simulink model "RC_Logitech_Mac"  (R2017b)
settings: Solver=FixedStepDiscrete  StartTime=0.0  StopTime=inf  RelTol=1e-3
libraries: vrlib x1
settings Model: Creator=zht  LastModifiedBy=zht

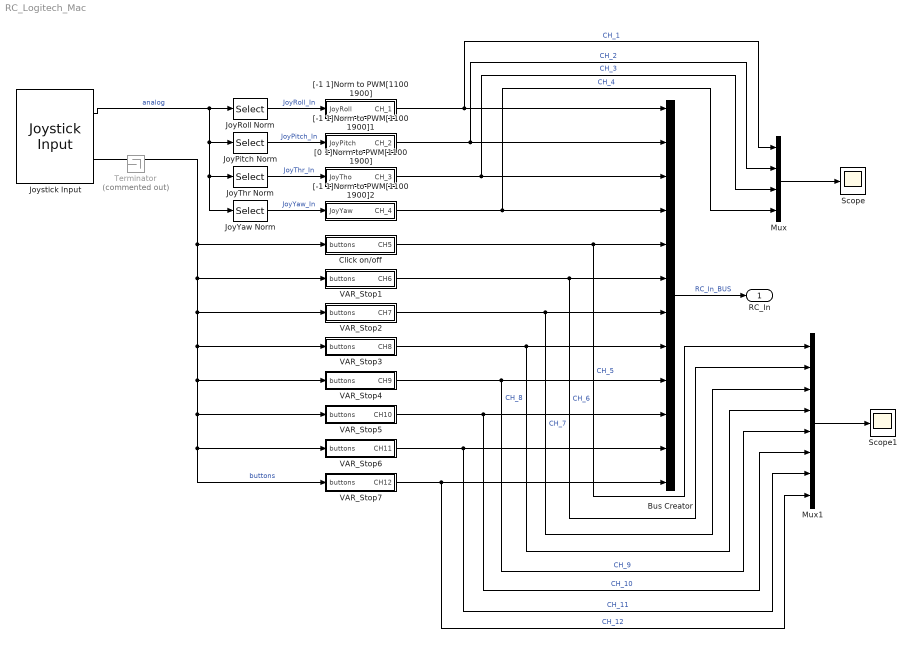
== system RC_Logitech_Mac ==
  Bus Creator : BusCreator  Inputs=12  OutDataTypeStr=Bus: RC_In_BUS  NonVirtualBus=on
  Click on/off : Subsystem
  JoyPitch Norm : Selector  InputPortWidth=4  IndexOptions=Index vector (dialog)  Indices=[2]  OutputSizes=1
  JoyRoll Norm : Selector  InputPortWidth=4  IndexOptions=Index vector (dialog)  Indices=[1]  OutputSizes=1
  JoyThr Norm : Selector  InputPortWidth=4  IndexOptions=Index vector (dialog)  Indices=[4]  OutputSizes=1
  JoyYaw Norm : Selector  InputPortWidth=4  IndexOptions=Index vector (dialog)  Indices=[3]  OutputSizes=1
  Joystick Input : vrlib/Joystick Input  joyid=1  adjustports=on  forcefeed=off
      settings: SourceProductBaseCode=VR
  Mux : Mux
  Mux1 : Mux  Inputs=8
  Scope : Scope
  Scope1 : Scope
  Terminator : Terminator  Commented=on
  VAR_Stop1 : Subsystem
  VAR_Stop2 : Subsystem
  VAR_Stop3 : Subsystem
  VAR_Stop4 : Subsystem
  VAR_Stop5 : Subsystem
  VAR_Stop6 : Subsystem
  VAR_Stop7 : Subsystem
  "[-1 1]Norm to PWM[1100 1900]" : Subsystem
  "[-1 1]Norm to PWM[1100 1900]1" : Subsystem
  "[-1 1]Norm to PWM[1100 1900]2" : Subsystem
  "[0 1]Norm to PWM[1100 1900]" : Subsystem
  RC_In : Outport  OutDataTypeStr=Bus: RC_In_BUS
  wires:
  Bus Creator/1 -> RC_In/1  "RC_In_BUS"
  JoyYaw Norm/1 -> "[-1 1]Norm to PWM[1100 1900]2"/1(JoyYaw)  "JoyYaw_In"
  JoyPitch Norm/1 -> "[-1 1]Norm to PWM[1100 1900]1"/1(JoyPitch)  "JoyPitch_In"
  "[0 1]Norm to PWM[1100 1900]"/1(CH_3) -> Bus Creator/3, Mux/3  "CH_3"
  Joystick Input/2 -> Click on/off/1(buttons), VAR_Stop1/1(buttons), VAR_Stop2/1(buttons), VAR_Stop3/1(buttons), VAR_Stop5/1(buttons), VAR_Stop6/1(buttons), VAR_Stop7/1(buttons), VAR_Stop4/1(buttons)  "buttons"
  Joystick Input/1 -> JoyYaw Norm/1, JoyThr Norm/1, JoyPitch Norm/1, JoyRoll Norm/1  "analog"
  "[-1 1]Norm to PWM[1100 1900]1"/1(CH_2) -> Bus Creator/2, Mux/2  "CH_2"
  "[-1 1]Norm to PWM[1100 1900]"/1(CH_1) -> Bus Creator/1, Mux/1  "CH_1"
  JoyThr Norm/1 -> "[0 1]Norm to PWM[1100 1900]"/1(JoyTho)  "JoyThr_In"
  JoyRoll Norm/1 -> "[-1 1]Norm to PWM[1100 1900]"/1(JoyRoll)  "JoyRoll_In"
  "[-1 1]Norm to PWM[1100 1900]2"/1(CH_4) -> Bus Creator/4, Mux/4  "CH_4"
  Click on/off/1(CH5) -> Bus Creator/5, Mux1/1  "CH_5"
  VAR_Stop1/1(CH6) -> Bus Creator/6, Mux1/2  "CH_6"
  VAR_Stop2/1(CH7) -> Bus Creator/7, Mux1/3  "CH_7"
  VAR_Stop3/1(CH8) -> Bus Creator/8, Mux1/4  "CH_8"
  VAR_Stop4/1(CH9) -> Bus Creator/9, Mux1/5  "CH_9"
  VAR_Stop5/1(CH10) -> Bus Creator/10, Mux1/6  "CH_10"
  VAR_Stop6/1(CH11) -> Bus Creator/11, Mux1/7  "CH_11"
  VAR_Stop7/1(CH12) -> Bus Creator/12, Mux1/8  "CH_12"
  Mux/1 -> Scope/1
  Mux1/1 -> Scope1/1

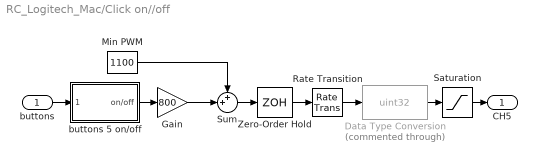
== system RC_Logitech_Mac/Click on//off ==
  buttons : Inport
  Data Type Conversion : DataTypeConversion  Commented=through  OutDataTypeStr=uint32
  Gain : Gain  Gain=800
  Min PWM : Constant  Value=1100
  Rate Transition : RateTransition
  Saturation : Saturate  UpperLimit=1900  LowerLimit=1100
  Sum : Sum  Inputs=++|
  Zero-Order Hold : ZeroOrderHold  SampleTime=0.02
  buttons 5 on/off : Subsystem
  CH5 : Outport
  wires:
  buttons/1 -> buttons 5 on/off/1(buttons)
  Min PWM/1 -> Sum/1
  Rate Transition/1 -> Data Type Conversion/1
  buttons 5 on/off/1(on/off) -> Gain/1
  Gain/1 -> Sum/2
  Data Type Conversion/1 -> Saturation/1
  Sum/1 -> Zero-Order Hold/1
  Zero-Order Hold/1 -> Rate Transition/1
  Saturation/1 -> CH5/1

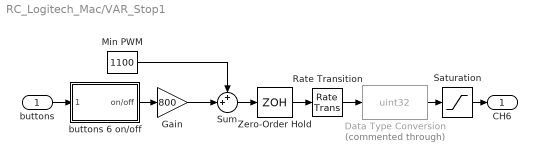
== system RC_Logitech_Mac/VAR_Stop1 ==
  buttons : Inport
  Data Type Conversion : DataTypeConversion  Commented=through  OutDataTypeStr=uint32
  Gain : Gain  Gain=800
  Min PWM : Constant  Value=1100
  Rate Transition : RateTransition
  Saturation : Saturate  UpperLimit=1900  LowerLimit=1100
  Sum : Sum  Inputs=++|
  Zero-Order Hold : ZeroOrderHold  SampleTime=0.02
  buttons 6 on/off : Subsystem
  CH6 : Outport
  wires:
  Saturation/1 -> CH6/1
  Zero-Order Hold/1 -> Rate Transition/1
  Sum/1 -> Zero-Order Hold/1
  Data Type Conversion/1 -> Saturation/1
  Gain/1 -> Sum/2
  buttons 6 on/off/1(on/off) -> Gain/1
  Rate Transition/1 -> Data Type Conversion/1
  Min PWM/1 -> Sum/1
  buttons/1 -> buttons 6 on/off/1(buttons)

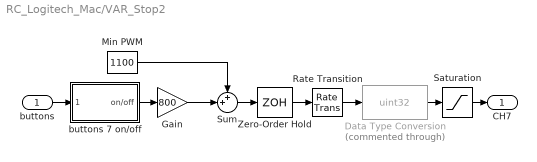
== system RC_Logitech_Mac/VAR_Stop2 ==
  buttons : Inport
  Data Type Conversion : DataTypeConversion  Commented=through  OutDataTypeStr=uint32
  Gain : Gain  Gain=800
  Min PWM : Constant  Value=1100
  Rate Transition : RateTransition
  Saturation : Saturate  UpperLimit=1900  LowerLimit=1100
  Sum : Sum  Inputs=++|
  Zero-Order Hold : ZeroOrderHold  SampleTime=0.02
  buttons 7 on/off : Subsystem
  CH7 : Outport
  wires:
  buttons/1 -> buttons 7 on/off/1(buttons)
  Min PWM/1 -> Sum/1
  Rate Transition/1 -> Data Type Conversion/1
  buttons 7 on/off/1(on/off) -> Gain/1
  Gain/1 -> Sum/2
  Data Type Conversion/1 -> Saturation/1
  Sum/1 -> Zero-Order Hold/1
  Zero-Order Hold/1 -> Rate Transition/1
  Saturation/1 -> CH7/1

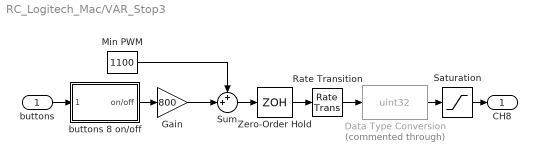
== system RC_Logitech_Mac/VAR_Stop3 ==
  buttons : Inport
  Data Type Conversion : DataTypeConversion  Commented=through  OutDataTypeStr=uint32
  Gain : Gain  Gain=800
  Min PWM : Constant  Value=1100
  Rate Transition : RateTransition
  Saturation : Saturate  UpperLimit=1900  LowerLimit=1100
  Sum : Sum  Inputs=++|
  Zero-Order Hold : ZeroOrderHold  SampleTime=0.02
  buttons 8 on/off : Subsystem
  CH8 : Outport
  wires:
  Saturation/1 -> CH8/1
  Zero-Order Hold/1 -> Rate Transition/1
  Sum/1 -> Zero-Order Hold/1
  Data Type Conversion/1 -> Saturation/1
  Gain/1 -> Sum/2
  buttons 8 on/off/1(on/off) -> Gain/1
  Rate Transition/1 -> Data Type Conversion/1
  Min PWM/1 -> Sum/1
  buttons/1 -> buttons 8 on/off/1(buttons)

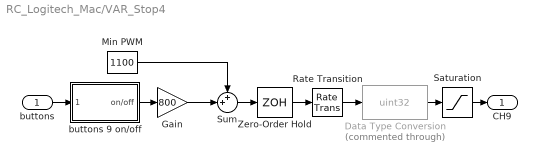
== system RC_Logitech_Mac/VAR_Stop4 ==
  buttons : Inport
  Data Type Conversion : DataTypeConversion  Commented=through  OutDataTypeStr=uint32
  Gain : Gain  Gain=800
  Min PWM : Constant  Value=1100
  Rate Transition : RateTransition
  Saturation : Saturate  UpperLimit=1900  LowerLimit=1100
  Sum : Sum  Inputs=++|
  Zero-Order Hold : ZeroOrderHold  SampleTime=0.02
  buttons 9 on/off : Subsystem
  CH9 : Outport
  wires:
  buttons/1 -> buttons 9 on/off/1(buttons)
  Min PWM/1 -> Sum/1
  Rate Transition/1 -> Data Type Conversion/1
  buttons 9 on/off/1(on/off) -> Gain/1
  Gain/1 -> Sum/2
  Data Type Conversion/1 -> Saturation/1
  Sum/1 -> Zero-Order Hold/1
  Zero-Order Hold/1 -> Rate Transition/1
  Saturation/1 -> CH9/1

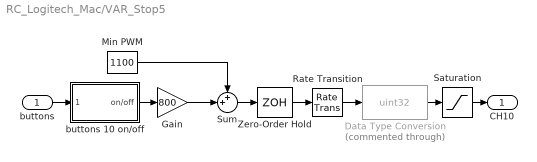
== system RC_Logitech_Mac/VAR_Stop5 ==
  buttons : Inport
  Data Type Conversion : DataTypeConversion  Commented=through  OutDataTypeStr=uint32
  Gain : Gain  Gain=800
  Min PWM : Constant  Value=1100
  Rate Transition : RateTransition
  Saturation : Saturate  UpperLimit=1900  LowerLimit=1100
  Sum : Sum  Inputs=++|
  Zero-Order Hold : ZeroOrderHold  SampleTime=0.02
  buttons 10 on/off : Subsystem
  CH10 : Outport
  wires:
  Saturation/1 -> CH10/1
  Zero-Order Hold/1 -> Rate Transition/1
  Sum/1 -> Zero-Order Hold/1
  Data Type Conversion/1 -> Saturation/1
  Gain/1 -> Sum/2
  buttons 10 on/off/1(on/off) -> Gain/1
  Rate Transition/1 -> Data Type Conversion/1
  Min PWM/1 -> Sum/1
  buttons/1 -> buttons 10 on/off/1(buttons)

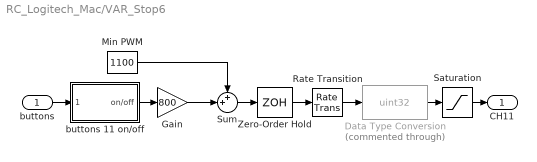
== system RC_Logitech_Mac/VAR_Stop6 ==
  buttons : Inport
  Data Type Conversion : DataTypeConversion  Commented=through  OutDataTypeStr=uint32
  Gain : Gain  Gain=800
  Min PWM : Constant  Value=1100
  Rate Transition : RateTransition
  Saturation : Saturate  UpperLimit=1900  LowerLimit=1100
  Sum : Sum  Inputs=++|
  Zero-Order Hold : ZeroOrderHold  SampleTime=0.02
  buttons 11 on/off : Subsystem
  CH11 : Outport
  wires:
  buttons/1 -> buttons 11 on/off/1(buttons)
  Min PWM/1 -> Sum/1
  Rate Transition/1 -> Data Type Conversion/1
  buttons 11 on/off/1(on/off) -> Gain/1
  Gain/1 -> Sum/2
  Data Type Conversion/1 -> Saturation/1
  Sum/1 -> Zero-Order Hold/1
  Zero-Order Hold/1 -> Rate Transition/1
  Saturation/1 -> CH11/1

== system RC_Logitech_Mac/VAR_Stop7 ==
  buttons : Inport
  Data Type Conversion : DataTypeConversion  Commented=through  OutDataTypeStr=uint32
  Gain : Gain  Gain=800
  Min PWM : Constant  Value=1100
  Rate Transition : RateTransition
  Saturation : Saturate  UpperLimit=1900  LowerLimit=1100
  Sum : Sum  Inputs=++|
  Zero-Order Hold : ZeroOrderHold  SampleTime=0.02
  buttons 12 on/off : Subsystem
  CH12 : Outport
  wires:
  Saturation/1 -> CH12/1
  Zero-Order Hold/1 -> Rate Transition/1
  Sum/1 -> Zero-Order Hold/1
  Data Type Conversion/1 -> Saturation/1
  Gain/1 -> Sum/2
  buttons 12 on/off/1(on/off) -> Gain/1
  Rate Transition/1 -> Data Type Conversion/1
  Min PWM/1 -> Sum/1
  buttons/1 -> buttons 12 on/off/1(buttons)

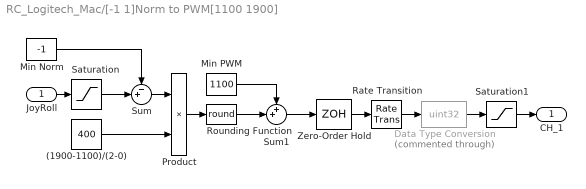
== system RC_Logitech_Mac/[-1 1]Norm to PWM[1100 1900] ==
  JoyRoll : Inport  OutDataTypeStr=double  Unit=1  PortDimensions=1
  (1900-1100)/(2-0) : Constant  Value=400  OutDataTypeStr=uint32
  Data Type Conversion : DataTypeConversion  Commented=through  OutDataTypeStr=uint32
  Min Norm : Constant  Value=-1
  Min PWM : Constant  Value=1100  OutDataTypeStr=uint32
  Product : Product  Inputs=**
  Rate Transition : RateTransition
  Rounding Function : Rounding  Operator=round
  Saturation : Saturate  UpperLimit=1  LowerLimit=-1
  Saturation1 : Saturate  UpperLimit=1900  LowerLimit=1100
  Sum : Sum  Inputs=-+|
  Sum1 : Sum  Inputs=++|
  Zero-Order Hold : ZeroOrderHold  SampleTime=0.02
  CH_1 : Outport  OutMin=[1100]  OutMax=[1900]  PortDimensions=1
  wires:
  JoyRoll/1 -> Saturation/1
  Saturation/1 -> Sum/2
  Min Norm/1 -> Sum/1
  Sum/1 -> Product/1
  (1900-1100)/(2-0)/1 -> Product/2
  Product/1 -> Rounding Function/1
  Min PWM/1 -> Sum1/1
  Sum1/1 -> Zero-Order Hold/1
  Rounding Function/1 -> Sum1/2
  Data Type Conversion/1 -> Saturation1/1
  Zero-Order Hold/1 -> Rate Transition/1
  Rate Transition/1 -> Data Type Conversion/1
  Saturation1/1 -> CH_1/1

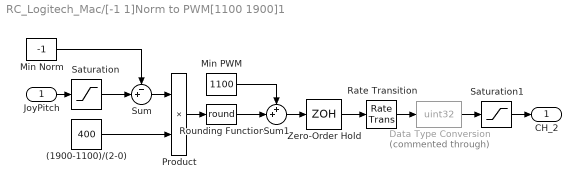
== system RC_Logitech_Mac/[-1 1]Norm to PWM[1100 1900]1 ==
  JoyPitch : Inport  OutDataTypeStr=double  Unit=1  PortDimensions=1
  (1900-1100)/(2-0) : Constant  Value=400
  Data Type Conversion : DataTypeConversion  Commented=through  OutDataTypeStr=uint32
  Min Norm : Constant  Value=-1
  Min PWM : Constant  Value=1100
  Product : Product  Inputs=**
  Rate Transition : RateTransition
  Rounding Function : Rounding  Operator=round
  Saturation : Saturate  UpperLimit=1  LowerLimit=-1
  Saturation1 : Saturate  UpperLimit=1900  LowerLimit=1100
  Sum : Sum  Inputs=-+|
  Sum1 : Sum  Inputs=++|
  Zero-Order Hold : ZeroOrderHold  SampleTime=0.02
  CH_2 : Outport  OutMin=[1100]  OutMax=[1900]  PortDimensions=1
  wires:
  Data Type Conversion/1 -> Saturation1/1
  Rounding Function/1 -> Sum1/2
  Min PWM/1 -> Sum1/1
  Product/1 -> Rounding Function/1
  (1900-1100)/(2-0)/1 -> Product/2
  Sum/1 -> Product/1
  Min Norm/1 -> Sum/1
  Saturation/1 -> Sum/2
  JoyPitch/1 -> Saturation/1
  Zero-Order Hold/1 -> Rate Transition/1
  Rate Transition/1 -> Data Type Conversion/1
  Saturation1/1 -> CH_2/1
  Sum1/1 -> Zero-Order Hold/1

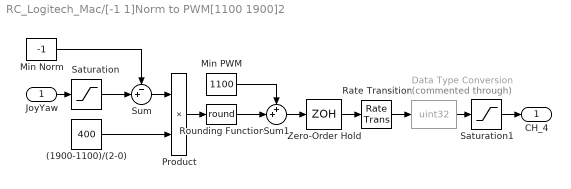
== system RC_Logitech_Mac/[-1 1]Norm to PWM[1100 1900]2 ==
  JoyYaw : Inport  OutDataTypeStr=double  Unit=1  PortDimensions=1
  (1900-1100)/(2-0) : Constant  Value=400
  Data Type Conversion : DataTypeConversion  Commented=through  OutDataTypeStr=uint32
  Min Norm : Constant  Value=-1
  Min PWM : Constant  Value=1100
  Product : Product  Inputs=**
  Rate Transition : RateTransition
  Rounding Function : Rounding  Operator=round
  Saturation : Saturate  UpperLimit=1  LowerLimit=-1
  Saturation1 : Saturate  UpperLimit=1900  LowerLimit=1100
  Sum : Sum  Inputs=-+|
  Sum1 : Sum  Inputs=++|
  Zero-Order Hold : ZeroOrderHold  SampleTime=0.02
  CH_4 : Outport  OutMin=[1100]  OutMax=[1900]  PortDimensions=1
  wires:
  JoyYaw/1 -> Saturation/1
  Saturation/1 -> Sum/2
  Min Norm/1 -> Sum/1
  Sum/1 -> Product/1
  (1900-1100)/(2-0)/1 -> Product/2
  Product/1 -> Rounding Function/1
  Min PWM/1 -> Sum1/1
  Sum1/1 -> Zero-Order Hold/1
  Rounding Function/1 -> Sum1/2
  Zero-Order Hold/1 -> Rate Transition/1
  Rate Transition/1 -> Data Type Conversion/1
  Data Type Conversion/1 -> Saturation1/1
  Saturation1/1 -> CH_4/1

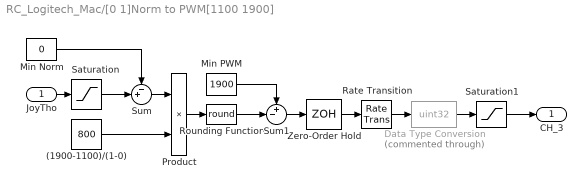
== system RC_Logitech_Mac/[0 1]Norm to PWM[1100 1900] ==
  JoyTho : Inport  OutDataTypeStr=double  Unit=1  PortDimensions=1
  (1900-1100)/(1-0) : Constant  Value=800
  Data Type Conversion : DataTypeConversion  Commented=through  OutDataTypeStr=uint32
  Min Norm : Constant  Value=0
  Min PWM : Constant  Value=1900
  Product : Product  Inputs=**
  Rate Transition : RateTransition
  Rounding Function : Rounding  Operator=round
  Saturation : Saturate  UpperLimit=1  LowerLimit=-1
  Saturation1 : Saturate  UpperLimit=1900  LowerLimit=1100
  Sum : Sum  Inputs=-+|
  Sum1 : Sum  Inputs=+-|
  Zero-Order Hold : ZeroOrderHold  SampleTime=0.02
  CH_3 : Outport  OutMin=[1100]  OutMax=[1900]  PortDimensions=1
  wires:
  JoyTho/1 -> Saturation/1
  Saturation/1 -> Sum/2
  Min Norm/1 -> Sum/1
  Sum/1 -> Product/1
  (1900-1100)/(1-0)/1 -> Product/2
  Product/1 -> Rounding Function/1
  Min PWM/1 -> Sum1/1
  Rounding Function/1 -> Sum1/2
  Zero-Order Hold/1 -> Rate Transition/1
  Rate Transition/1 -> Data Type Conversion/1
  Data Type Conversion/1 -> Saturation1/1
  Sum1/1 -> Zero-Order Hold/1
  Saturation1/1 -> CH_3/1

== system RC_Logitech_Mac/Click on//off/buttons 5 on//off ==
  buttons : Inport
  Selector : Selector  InputPortWidth=12  IndexOptions=Index vector (dialog)  Indices=[5]  OutputSizes=1
  on/off : Outport  OutDataTypeStr=boolean  PortDimensions=1
  wires:
  Selector/1 -> on/off/1
  buttons/1 -> Selector/1

== system RC_Logitech_Mac/VAR_Stop1/buttons 6 on//off ==
  buttons : Inport
  Selector : Selector  InputPortWidth=12  IndexOptions=Index vector (dialog)  Indices=[6]  OutputSizes=1
  on/off : Outport  OutDataTypeStr=boolean  PortDimensions=1
  wires:
  buttons/1 -> Selector/1
  Selector/1 -> on/off/1

== system RC_Logitech_Mac/VAR_Stop2/buttons 7 on//off ==
  buttons : Inport
  Selector : Selector  InputPortWidth=12  IndexOptions=Index vector (dialog)  Indices=[7]  OutputSizes=1
  on/off : Outport  OutDataTypeStr=boolean  PortDimensions=1
  wires:
  buttons/1 -> Selector/1
  Selector/1 -> on/off/1

== system RC_Logitech_Mac/VAR_Stop3/buttons 8 on//off ==
  buttons : Inport
  Selector : Selector  InputPortWidth=12  IndexOptions=Index vector (dialog)  Indices=[8]  OutputSizes=1
  on/off : Outport  OutDataTypeStr=boolean  PortDimensions=1
  wires:
  buttons/1 -> Selector/1
  Selector/1 -> on/off/1

== system RC_Logitech_Mac/VAR_Stop4/buttons 9 on//off ==
  buttons : Inport
  Selector : Selector  InputPortWidth=12  IndexOptions=Index vector (dialog)  Indices=[9]  OutputSizes=1
  on/off : Outport  OutDataTypeStr=boolean  PortDimensions=1
  wires:
  buttons/1 -> Selector/1
  Selector/1 -> on/off/1

== system RC_Logitech_Mac/VAR_Stop5/buttons 10 on//off ==
  buttons : Inport
  Selector : Selector  InputPortWidth=12  IndexOptions=Index vector (dialog)  Indices=[10]  OutputSizes=1
  on/off : Outport  OutDataTypeStr=boolean  PortDimensions=1
  wires:
  buttons/1 -> Selector/1
  Selector/1 -> on/off/1

== system RC_Logitech_Mac/VAR_Stop6/buttons 11 on//off ==
  buttons : Inport
  Selector : Selector  InputPortWidth=12  IndexOptions=Index vector (dialog)  Indices=[11]  OutputSizes=1
  on/off : Outport  OutDataTypeStr=boolean  PortDimensions=1
  wires:
  buttons/1 -> Selector/1
  Selector/1 -> on/off/1

== system RC_Logitech_Mac/VAR_Stop7/buttons 12 on//off ==
  buttons : Inport
  Selector : Selector  InputPortWidth=12  IndexOptions=Index vector (dialog)  Indices=[12]  OutputSizes=1
  on/off : Outport  OutDataTypeStr=boolean  PortDimensions=1
  wires:
  buttons/1 -> Selector/1
  Selector/1 -> on/off/1
